simulink model "generic_src"  (Simulink 10.3)
settings: Solver=ode45  StartTime=0.0  StopTime=inf  RelTol=1e-3  EnableMultiTasking=on
undefined symbols (not defined in the file or in its folder): Area_Front, Area_Rear, ay_max_off, ay_max_on, ay_per_mu_max_off, ay_per_mu_max_on, Brake_ratio, brake_valve_ctrl_kP, cat1mode1_higher, cat1mode1_lower, cat1mode2_higher, cat1mode2_lower, cat1mode3_higher, cat1mode3_lower, cat2mode1_higher, cat2mode1_lower, cat2mode2_higher, cat2mode2_lower, cat2mode3_higher, cat2mode3_lower, delta_vel, diff_lock_fac, diff_lock_off, diff_lock_on, ESP_ctrl_kD, ESP_ctrl_kI, ESP_ctrl_kP, ESP_ctrl_restore_kI, ESP_min_throttle_fac, f_ax, f_slip, g, higherlimit_highvel, higherlimit_lowvel, highervel_fac, highervelocity_fac, InitialConditionForIntegrator, limit_acc, limit_selectlow, limit_starting, limit_vdiff, locktime_throttle, lowerlimit_highvel, lowerlimit_lowvel, lowervel_fac, lowervelocity_fac, min_throttle, MPS2KMPH, MSR_ctrl_kD, MSR_ctrl_kI, MSR_ctrl_kP, MSR_min_throttle_fac, PID_kP_sideslip, PID_kP_yawrate, RADpS2RpM, rBrake, RpM2RADpS, SH_SL_switch, sideslip_vel_corr, sidesplip_deviation_max ... (+35)
libraries: CarMaker4SL x137, simulink x57, simulink_extras x6
(part 7 of 12)

== system generic_src/CarMaker/IPG Vehicle/PowerTrain/PTControl Example/PTControl_In/CreateBus PTC_Cfg Gearbox8 ==
  In : Inport
  BusCreator : BusCreator  Inputs=38
  Demux : Demux  Outputs=38
      settings: DisplayOption=none
  Out : Outport  VectorParamsAs1DForOutWhenUnconnected=off
  wires:
  Demux/38 -> BusCreator/38  "PTC_Cfg Gearbox8 iBGear16"
  Demux/37 -> BusCreator/37  "PTC_Cfg Gearbox8 iBGear15"
  Demux/36 -> BusCreator/36  "PTC_Cfg Gearbox8 iBGear14"
  Demux/35 -> BusCreator/35  "PTC_Cfg Gearbox8 iBGear13"
  Demux/34 -> BusCreator/34  "PTC_Cfg Gearbox8 iBGear12"
  Demux/33 -> BusCreator/33  "PTC_Cfg Gearbox8 iBGear11"
  Demux/32 -> BusCreator/32  "PTC_Cfg Gearbox8 iBGear10"
  Demux/31 -> BusCreator/31  "PTC_Cfg Gearbox8 iBGear9"
  Demux/30 -> BusCreator/30  "PTC_Cfg Gearbox8 iBGear8"
  Demux/29 -> BusCreator/29  "PTC_Cfg Gearbox8 iBGear7"
  Demux/28 -> BusCreator/28  "PTC_Cfg Gearbox8 iBGear6"
  Demux/27 -> BusCreator/27  "PTC_Cfg Gearbox8 iBGear5"
  Demux/26 -> BusCreator/26  "PTC_Cfg Gearbox8 iBGear4"
  Demux/25 -> BusCreator/25  "PTC_Cfg Gearbox8 iBGear3"
  Demux/24 -> BusCreator/24  "PTC_Cfg Gearbox8 iBGear2"
  Demux/23 -> BusCreator/23  "PTC_Cfg Gearbox8 iBGear1"
  Demux/22 -> BusCreator/22  "PTC_Cfg Gearbox8 iBGear0"
  Demux/21 -> BusCreator/21  "PTC_Cfg Gearbox8 nBGears"
  Demux/20 -> BusCreator/20  "PTC_Cfg Gearbox8 iFGear16"
  Demux/19 -> BusCreator/19  "PTC_Cfg Gearbox8 iFGear15"
  Demux/18 -> BusCreator/18  "PTC_Cfg Gearbox8 iFGear14"
  Demux/17 -> BusCreator/17  "PTC_Cfg Gearbox8 iFGear13"
  Demux/16 -> BusCreator/16  "PTC_Cfg Gearbox8 iFGear12"
  Demux/15 -> BusCreator/15  "PTC_Cfg Gearbox8 iFGear11"
  Demux/14 -> BusCreator/14  "PTC_Cfg Gearbox8 iFGear10"
  Demux/13 -> BusCreator/13  "PTC_Cfg Gearbox8 iFGear9"
  Demux/12 -> BusCreator/12  "PTC_Cfg Gearbox8 iFGear8"
  Demux/11 -> BusCreator/11  "PTC_Cfg Gearbox8 iFGear7"
  Demux/10 -> BusCreator/10  "PTC_Cfg Gearbox8 iFGear6"
  Demux/9 -> BusCreator/9  "PTC_Cfg Gearbox8 iFGear5"
  Demux/8 -> BusCreator/8  "PTC_Cfg Gearbox8 iFGear4"
  Demux/7 -> BusCreator/7  "PTC_Cfg Gearbox8 iFGear3"
  Demux/6 -> BusCreator/6  "PTC_Cfg Gearbox8 iFGear2"
  Demux/5 -> BusCreator/5  "PTC_Cfg Gearbox8 iFGear1"
  Demux/4 -> BusCreator/4  "PTC_Cfg Gearbox8 iFGear0"
  Demux/3 -> BusCreator/3  "PTC_Cfg Gearbox8 nFGears"
  Demux/2 -> BusCreator/2  "PTC_Cfg Gearbox8 ClKind"
  Demux/1 -> BusCreator/1  "PTC_Cfg Gearbox8 GBKind"
  BusCreator/1 -> Out/1
  In/1 -> Demux/1

== system generic_src/CarMaker/IPG Vehicle/PowerTrain/PTControl Example/PTControl_In/CreateBus PTC_Cfg Gearbox9 ==
  In : Inport
  BusCreator : BusCreator  Inputs=38
  Demux : Demux  Outputs=38
      settings: DisplayOption=none
  Out : Outport  VectorParamsAs1DForOutWhenUnconnected=off
  wires:
  Demux/38 -> BusCreator/38  "PTC_Cfg Gearbox9 iBGear16"
  Demux/37 -> BusCreator/37  "PTC_Cfg Gearbox9 iBGear15"
  Demux/36 -> BusCreator/36  "PTC_Cfg Gearbox9 iBGear14"
  Demux/35 -> BusCreator/35  "PTC_Cfg Gearbox9 iBGear13"
  Demux/34 -> BusCreator/34  "PTC_Cfg Gearbox9 iBGear12"
  Demux/33 -> BusCreator/33  "PTC_Cfg Gearbox9 iBGear11"
  Demux/32 -> BusCreator/32  "PTC_Cfg Gearbox9 iBGear10"
  Demux/31 -> BusCreator/31  "PTC_Cfg Gearbox9 iBGear9"
  Demux/30 -> BusCreator/30  "PTC_Cfg Gearbox9 iBGear8"
  Demux/29 -> BusCreator/29  "PTC_Cfg Gearbox9 iBGear7"
  Demux/28 -> BusCreator/28  "PTC_Cfg Gearbox9 iBGear6"
  Demux/27 -> BusCreator/27  "PTC_Cfg Gearbox9 iBGear5"
  Demux/26 -> BusCreator/26  "PTC_Cfg Gearbox9 iBGear4"
  Demux/25 -> BusCreator/25  "PTC_Cfg Gearbox9 iBGear3"
  Demux/24 -> BusCreator/24  "PTC_Cfg Gearbox9 iBGear2"
  Demux/23 -> BusCreator/23  "PTC_Cfg Gearbox9 iBGear1"
  Demux/22 -> BusCreator/22  "PTC_Cfg Gearbox9 iBGear0"
  Demux/21 -> BusCreator/21  "PTC_Cfg Gearbox9 nBGears"
  Demux/20 -> BusCreator/20  "PTC_Cfg Gearbox9 iFGear16"
  Demux/19 -> BusCreator/19  "PTC_Cfg Gearbox9 iFGear15"
  Demux/18 -> BusCreator/18  "PTC_Cfg Gearbox9 iFGear14"
  Demux/17 -> BusCreator/17  "PTC_Cfg Gearbox9 iFGear13"
  Demux/16 -> BusCreator/16  "PTC_Cfg Gearbox9 iFGear12"
  Demux/15 -> BusCreator/15  "PTC_Cfg Gearbox9 iFGear11"
  Demux/14 -> BusCreator/14  "PTC_Cfg Gearbox9 iFGear10"
  Demux/13 -> BusCreator/13  "PTC_Cfg Gearbox9 iFGear9"
  Demux/12 -> BusCreator/12  "PTC_Cfg Gearbox9 iFGear8"
  Demux/11 -> BusCreator/11  "PTC_Cfg Gearbox9 iFGear7"
  Demux/10 -> BusCreator/10  "PTC_Cfg Gearbox9 iFGear6"
  Demux/9 -> BusCreator/9  "PTC_Cfg Gearbox9 iFGear5"
  Demux/8 -> BusCreator/8  "PTC_Cfg Gearbox9 iFGear4"
  Demux/7 -> BusCreator/7  "PTC_Cfg Gearbox9 iFGear3"
  Demux/6 -> BusCreator/6  "PTC_Cfg Gearbox9 iFGear2"
  Demux/5 -> BusCreator/5  "PTC_Cfg Gearbox9 iFGear1"
  Demux/4 -> BusCreator/4  "PTC_Cfg Gearbox9 iFGear0"
  Demux/3 -> BusCreator/3  "PTC_Cfg Gearbox9 nFGears"
  Demux/2 -> BusCreator/2  "PTC_Cfg Gearbox9 ClKind"
  Demux/1 -> BusCreator/1  "PTC_Cfg Gearbox9 GBKind"
  BusCreator/1 -> Out/1
  In/1 -> Demux/1

== system generic_src/CarMaker/IPG Vehicle/PowerTrain/PTControl Example/PTControl_In/CreateBus PTC_Cfg ISG ==
  In : Inport
  BusCreator : BusCreator  Inputs=4
  Demux : Demux
      settings: DisplayOption=none
  Out : Outport  VectorParamsAs1DForOutWhenUnconnected=off
  wires:
  Demux/4 -> BusCreator/4  "PTC_Cfg ISG rotv_Gen_max"
  Demux/3 -> BusCreator/3  "PTC_Cfg ISG rotv_Mot_max"
  Demux/2 -> BusCreator/2  "PTC_Cfg ISG Ratio"
  Demux/1 -> BusCreator/1  "PTC_Cfg ISG Level"
  BusCreator/1 -> Out/1
  In/1 -> Demux/1

== system generic_src/CarMaker/IPG Vehicle/PowerTrain/PTControl Example/PTControl_In/CreateBus PTC_Cfg Misc ==
  In : Inport
  BusCreator : BusCreator  Inputs=14
  Demux : Demux  Outputs=14
      settings: DisplayOption=none
  Out : Outport  VectorParamsAs1DForOutWhenUnconnected=off
  wires:
  BusCreator/1 -> Out/1
  In/1 -> Demux/1
  Demux/4 -> BusCreator/4  "PTC_Cfg nClutch"
  Demux/11 -> BusCreator/11  "PTC_Cfg DriveSourcePos0"
  Demux/12 -> BusCreator/12  "PTC_Cfg DriveSourcePos1"
  Demux/14 -> BusCreator/14  "PTC_Cfg DriveSourcePos3"
  Demux/5 -> BusCreator/5  "PTC_Cfg nGearbox"
  Demux/2 -> BusCreator/2  "PTC_Cfg ClKind"
  Demux/10 -> BusCreator/10  "PTC_Cfg DL_iDiff_mean"
  Demux/9 -> BusCreator/9  "PTC_Cfg Aero_Frcx"
  Demux/1 -> BusCreator/1  "PTC_Cfg PTKind"
  Demux/8 -> BusCreator/8  "PTC_Cfg WheelRadius"
  Demux/13 -> BusCreator/13  "PTC_Cfg DriveSourcePos2"
  Demux/7 -> BusCreator/7  "PTC_Cfg Vehicle_nWheels"
  Demux/3 -> BusCreator/3  "PTC_Cfg nMotor"
  Demux/6 -> BusCreator/6  "PTC_Cfg nPlanetGear"

== system generic_src/CarMaker/IPG Vehicle/PowerTrain/PTControl Example/PTControl_In/CreateBus PTC_Cfg Motor ==
  In : Inport
  BusCreator : BusCreator  Inputs=48
  Demux : Demux  Outputs=48
      settings: DisplayOption=none
  Out : Outport  VectorParamsAs1DForOutWhenUnconnected=off
  wires:
  Demux/16 -> BusCreator/16  "PTC_Cfg Motor3 rotv_Gen_max"
  Demux/15 -> BusCreator/15  "PTC_Cfg Motor3 rotv_Mot_max"
  Demux/14 -> BusCreator/14  "PTC_Cfg Motor3 Ratio"
  Demux/13 -> BusCreator/13  "PTC_Cfg Motor3 Level"
  Demux/12 -> BusCreator/12  "PTC_Cfg Motor2 rotv_Gen_max"
  Demux/11 -> BusCreator/11  "PTC_Cfg Motor2 rotv_Mot_max"
  Demux/10 -> BusCreator/10  "PTC_Cfg Motor2 Ratio"
  Demux/9 -> BusCreator/9  "PTC_Cfg Motor2 Level"
  Demux/8 -> BusCreator/8  "PTC_Cfg Motor1 rotv_Gen_max"
  Demux/7 -> BusCreator/7  "PTC_Cfg Motor1 rotv_Mot_max"
  Demux/6 -> BusCreator/6  "PTC_Cfg Motor1 Ratio"
  Demux/5 -> BusCreator/5  "PTC_Cfg Motor1 Level"
  Demux/4 -> BusCreator/4  "PTC_Cfg Motor0 rotv_Gen_max"
  Demux/3 -> BusCreator/3  "PTC_Cfg Motor0 rotv_Mot_max"
  Demux/2 -> BusCreator/2  "PTC_Cfg Motor0 Ratio"
  Demux/1 -> BusCreator/1  "PTC_Cfg Motor0 Level"
  BusCreator/1 -> Out/1
  In/1 -> Demux/1
  Demux/17 -> BusCreator/17  "PTC_Cfg Motor4 Level"
  Demux/18 -> BusCreator/18  "PTC_Cfg Motor4 Ratio"
  Demux/19 -> BusCreator/19  "PTC_Cfg Motor4 rotv_Mot_max"
  Demux/20 -> BusCreator/20  "PTC_Cfg Motor4 rotv_Gen_max"
  Demux/21 -> BusCreator/21  "PTC_Cfg Motor5 Level"
  Demux/22 -> BusCreator/22  "PTC_Cfg Motor5 Ratio"
  Demux/23 -> BusCreator/23  "PTC_Cfg Motor5 rotv_Mot_max"
  Demux/24 -> BusCreator/24  "PTC_Cfg Motor5 rotv_Gen_max"
  Demux/25 -> BusCreator/25  "PTC_Cfg Motor6 Level"
  Demux/26 -> BusCreator/26  "PTC_Cfg Motor6 Ratio"
  Demux/27 -> BusCreator/27  "PTC_Cfg Motor6 rotv_Mot_max"
  Demux/28 -> BusCreator/28  "PTC_Cfg Motor6 rotv_Gen_max"
  Demux/29 -> BusCreator/29  "PTC_Cfg Motor7 Level"
  Demux/30 -> BusCreator/30  "PTC_Cfg Motor7 Ratio"
  Demux/31 -> BusCreator/31  "PTC_Cfg Motor7 rotv_Mot_max"
  Demux/32 -> BusCreator/32  "PTC_Cfg Motor7 rotv_Gen_max"
  Demux/33 -> BusCreator/33  "PTC_Cfg Motor8 Level"
  Demux/34 -> BusCreator/34  "PTC_Cfg Motor8 Ratio"
  Demux/35 -> BusCreator/35  "PTC_Cfg Motor8 rotv_Mot_max"
  Demux/36 -> BusCreator/36  "PTC_Cfg Motor8 rotv_Gen_max"
  Demux/37 -> BusCreator/37  "PTC_Cfg Motor9 Level"
  Demux/38 -> BusCreator/38  "PTC_Cfg Motor9 Ratio"
  Demux/39 -> BusCreator/39  "PTC_Cfg Motor9 rotv_Mot_max"
  Demux/40 -> BusCreator/40  "PTC_Cfg Motor9 rotv_Gen_max"
  Demux/41 -> BusCreator/41  "PTC_Cfg Motor10 Level"
  Demux/42 -> BusCreator/42  "PTC_Cfg Motor10 Ratio"
  Demux/43 -> BusCreator/43  "PTC_Cfg Motor10 rotv_Mot_max"
  Demux/44 -> BusCreator/44  "PTC_Cfg Motor10 rotv_Gen_max"
  Demux/45 -> BusCreator/45  "PTC_Cfg Motor11 Level"
  Demux/46 -> BusCreator/46  "PTC_Cfg Motor11 Ratio"
  Demux/47 -> BusCreator/47  "PTC_Cfg Motor11 rotv_Mot_max"
  Demux/48 -> BusCreator/48  "PTC_Cfg Motor11 rotv_Gen_max"

== system generic_src/CarMaker/IPG Vehicle/PowerTrain/PTControl Example/PTControl_In/CreateBus PTC_Cfg PlanetGear ==
  In : Inport
  BusCreator : BusCreator  Inputs=1
  Demux : Demux  Outputs=1
      settings: DisplayOption=none
  Out : Outport  VectorParamsAs1DForOutWhenUnconnected=off
  wires:
  Demux/1 -> BusCreator/1  "PTC_Cfg PlanetGear0 Ratio"
  BusCreator/1 -> Out/1
  In/1 -> Demux/1

== system generic_src/CarMaker/IPG Vehicle/PowerTrain/TCU Example/PTTransmCU_In/CreateBus TCU ClutchIn0 ==
  In : Inport
  BusCreator : BusCreator  Inputs=7
  Demux : Demux  Outputs=7
      settings: DisplayOption=none
  Out : Outport  VectorParamsAs1DForOutWhenUnconnected=off
  wires:
  Demux/7 -> BusCreator/7  "TCU ClutchIn0 i_TrqIn2Out"
  Demux/6 -> BusCreator/6  "TCU ClutchIn0 Trq_out_trg"
  Demux/5 -> BusCreator/5  "TCU ClutchIn0 Trq_out"
  Demux/4 -> BusCreator/4  "TCU ClutchIn0 Trq_in"
  Demux/3 -> BusCreator/3  "TCU ClutchIn0 rotv_out_trg"
  Demux/2 -> BusCreator/2  "TCU ClutchIn0 rotv_out"
  Demux/1 -> BusCreator/1  "TCU ClutchIn0 rotv_in"
  BusCreator/1 -> Out/1
  In/1 -> Demux/1

== system generic_src/CarMaker/IPG Vehicle/PowerTrain/TCU Example/PTTransmCU_In/CreateBus TCU ClutchIn1 ==
  In : Inport
  BusCreator : BusCreator  Inputs=7
  Demux : Demux  Outputs=7
      settings: DisplayOption=none
  Out : Outport  VectorParamsAs1DForOutWhenUnconnected=off
  wires:
  Demux/7 -> BusCreator/7  "TCU ClutchIn1 i_TrqIn2Out"
  Demux/6 -> BusCreator/6  "TCU ClutchIn1 Trq_out_trg"
  Demux/5 -> BusCreator/5  "TCU ClutchIn1 Trq_out"
  Demux/4 -> BusCreator/4  "TCU ClutchIn1 Trq_in"
  Demux/3 -> BusCreator/3  "TCU ClutchIn1 rotv_out_trg"
  Demux/2 -> BusCreator/2  "TCU ClutchIn1 rotv_out"
  Demux/1 -> BusCreator/1  "TCU ClutchIn1 rotv_in"
  BusCreator/1 -> Out/1
  In/1 -> Demux/1

== system generic_src/CarMaker/IPG Vehicle/PowerTrain/TCU Example/PTTransmCU_In/CreateBus TCU ClutchIn10 ==
  In : Inport
  BusCreator : BusCreator  Inputs=7
  Demux : Demux  Outputs=7
      settings: DisplayOption=none
  Out : Outport  VectorParamsAs1DForOutWhenUnconnected=off
  wires:
  Demux/7 -> BusCreator/7  "TCU ClutchIn10 i_TrqIn2Out"
  Demux/6 -> BusCreator/6  "TCU ClutchIn10 Trq_out_trg"
  Demux/5 -> BusCreator/5  "TCU ClutchIn10 Trq_out"
  Demux/4 -> BusCreator/4  "TCU ClutchIn10 Trq_in"
  Demux/3 -> BusCreator/3  "TCU ClutchIn10 rotv_out_trg"
  Demux/2 -> BusCreator/2  "TCU ClutchIn10 rotv_out"
  Demux/1 -> BusCreator/1  "TCU ClutchIn10 rotv_in"
  BusCreator/1 -> Out/1
  In/1 -> Demux/1

== system generic_src/CarMaker/IPG Vehicle/PowerTrain/TCU Example/PTTransmCU_In/CreateBus TCU ClutchIn11 ==
  In : Inport
  BusCreator : BusCreator  Inputs=7
  Demux : Demux  Outputs=7
      settings: DisplayOption=none
  Out : Outport  VectorParamsAs1DForOutWhenUnconnected=off
  wires:
  Demux/7 -> BusCreator/7  "TCU ClutchIn10 i_TrqIn2Out"
  Demux/6 -> BusCreator/6  "TCU ClutchIn10 Trq_out_trg"
  Demux/5 -> BusCreator/5  "TCU ClutchIn10 Trq_out"
  Demux/4 -> BusCreator/4  "TCU ClutchIn10 Trq_in"
  Demux/3 -> BusCreator/3  "TCU ClutchIn10 rotv_out_trg"
  Demux/2 -> BusCreator/2  "TCU ClutchIn10 rotv_out"
  Demux/1 -> BusCreator/1  "TCU ClutchIn10 rotv_in"
  BusCreator/1 -> Out/1
  In/1 -> Demux/1

== system generic_src/CarMaker/IPG Vehicle/PowerTrain/TCU Example/PTTransmCU_In/CreateBus TCU ClutchIn2 ==
  In : Inport
  BusCreator : BusCreator  Inputs=7
  Demux : Demux  Outputs=7
      settings: DisplayOption=none
  Out : Outport  VectorParamsAs1DForOutWhenUnconnected=off
  wires:
  Demux/7 -> BusCreator/7  "TCU ClutchIn2 i_TrqIn2Out"
  Demux/6 -> BusCreator/6  "TCU ClutchIn2 Trq_out_trg"
  Demux/5 -> BusCreator/5  "TCU ClutchIn2 Trq_out"
  Demux/4 -> BusCreator/4  "TCU ClutchIn2 Trq_in"
  Demux/3 -> BusCreator/3  "TCU ClutchIn2 rotv_out_trg"
  Demux/2 -> BusCreator/2  "TCU ClutchIn2 rotv_out"
  Demux/1 -> BusCreator/1  "TCU ClutchIn2 rotv_in"
  BusCreator/1 -> Out/1
  In/1 -> Demux/1

== system generic_src/CarMaker/IPG Vehicle/PowerTrain/TCU Example/PTTransmCU_In/CreateBus TCU ClutchIn3 ==
  In : Inport
  BusCreator : BusCreator  Inputs=7
  Demux : Demux  Outputs=7
      settings: DisplayOption=none
  Out : Outport  VectorParamsAs1DForOutWhenUnconnected=off
  wires:
  Demux/7 -> BusCreator/7  "TCU ClutchIn3 i_TrqIn2Out"
  Demux/6 -> BusCreator/6  "TCU ClutchIn3 Trq_out_trg"
  Demux/5 -> BusCreator/5  "TCU ClutchIn3 Trq_out"
  Demux/4 -> BusCreator/4  "TCU ClutchIn3 Trq_in"
  Demux/3 -> BusCreator/3  "TCU ClutchIn3 rotv_out_trg"
  Demux/2 -> BusCreator/2  "TCU ClutchIn3 rotv_out"
  Demux/1 -> BusCreator/1  "TCU ClutchIn3 rotv_in"
  BusCreator/1 -> Out/1
  In/1 -> Demux/1

== system generic_src/CarMaker/IPG Vehicle/PowerTrain/TCU Example/PTTransmCU_In/CreateBus TCU ClutchIn4 ==
  In : Inport
  BusCreator : BusCreator  Inputs=7
  Demux : Demux  Outputs=7
      settings: DisplayOption=none
  Out : Outport  VectorParamsAs1DForOutWhenUnconnected=off
  wires:
  Demux/7 -> BusCreator/7  "TCU ClutchIn4 i_TrqIn2Out"
  Demux/6 -> BusCreator/6  "TCU ClutchIn4 Trq_out_trg"
  Demux/5 -> BusCreator/5  "TCU ClutchIn4 Trq_out"
  Demux/4 -> BusCreator/4  "TCU ClutchIn4 Trq_in"
  Demux/3 -> BusCreator/3  "TCU ClutchIn4 rotv_out_trg"
  Demux/2 -> BusCreator/2  "TCU ClutchIn4 rotv_out"
  Demux/1 -> BusCreator/1  "TCU ClutchIn4 rotv_in"
  BusCreator/1 -> Out/1
  In/1 -> Demux/1

== system generic_src/CarMaker/IPG Vehicle/PowerTrain/TCU Example/PTTransmCU_In/CreateBus TCU ClutchIn5 ==
  In : Inport
  BusCreator : BusCreator  Inputs=7
  Demux : Demux  Outputs=7
      settings: DisplayOption=none
  Out : Outport  VectorParamsAs1DForOutWhenUnconnected=off
  wires:
  Demux/7 -> BusCreator/7  "TCU ClutchIn5 i_TrqIn2Out"
  Demux/6 -> BusCreator/6  "TCU ClutchIn5 Trq_out_trg"
  Demux/5 -> BusCreator/5  "TCU ClutchIn5 Trq_out"
  Demux/4 -> BusCreator/4  "TCU ClutchIn5 Trq_in"
  Demux/3 -> BusCreator/3  "TCU ClutchIn5 rotv_out_trg"
  Demux/2 -> BusCreator/2  "TCU ClutchIn5 rotv_out"
  Demux/1 -> BusCreator/1  "TCU ClutchIn5 rotv_in"
  BusCreator/1 -> Out/1
  In/1 -> Demux/1

== system generic_src/CarMaker/IPG Vehicle/PowerTrain/TCU Example/PTTransmCU_In/CreateBus TCU ClutchIn6 ==
  In : Inport
  BusCreator : BusCreator  Inputs=7
  Demux : Demux  Outputs=7
      settings: DisplayOption=none
  Out : Outport  VectorParamsAs1DForOutWhenUnconnected=off
  wires:
  Demux/7 -> BusCreator/7  "TCU ClutchIn6 i_TrqIn2Out"
  Demux/6 -> BusCreator/6  "TCU ClutchIn6 Trq_out_trg"
  Demux/5 -> BusCreator/5  "TCU ClutchIn6 Trq_out"
  Demux/4 -> BusCreator/4  "TCU ClutchIn6 Trq_in"
  Demux/3 -> BusCreator/3  "TCU ClutchIn6 rotv_out_trg"
  Demux/2 -> BusCreator/2  "TCU ClutchIn6 rotv_out"
  Demux/1 -> BusCreator/1  "TCU ClutchIn6 rotv_in"
  BusCreator/1 -> Out/1
  In/1 -> Demux/1

== system generic_src/CarMaker/IPG Vehicle/PowerTrain/TCU Example/PTTransmCU_In/CreateBus TCU ClutchIn7 ==
  In : Inport
  BusCreator : BusCreator  Inputs=7
  Demux : Demux  Outputs=7
      settings: DisplayOption=none
  Out : Outport  VectorParamsAs1DForOutWhenUnconnected=off
  wires:
  Demux/7 -> BusCreator/7  "TCU ClutchIn7 i_TrqIn2Out"
  Demux/6 -> BusCreator/6  "TCU ClutchIn7 Trq_out_trg"
  Demux/5 -> BusCreator/5  "TCU ClutchIn7 Trq_out"
  Demux/4 -> BusCreator/4  "TCU ClutchIn7 Trq_in"
  Demux/3 -> BusCreator/3  "TCU ClutchIn7 rotv_out_trg"
  Demux/2 -> BusCreator/2  "TCU ClutchIn7 rotv_out"
  Demux/1 -> BusCreator/1  "TCU ClutchIn7 rotv_in"
  BusCreator/1 -> Out/1
  In/1 -> Demux/1

== system generic_src/CarMaker/IPG Vehicle/PowerTrain/TCU Example/PTTransmCU_In/CreateBus TCU ClutchIn8 ==
  In : Inport
  BusCreator : BusCreator  Inputs=7
  Demux : Demux  Outputs=7
      settings: DisplayOption=none
  Out : Outport  VectorParamsAs1DForOutWhenUnconnected=off
  wires:
  Demux/7 -> BusCreator/7  "TCU ClutchIn8 i_TrqIn2Out"
  Demux/6 -> BusCreator/6  "TCU ClutchIn8 Trq_out_trg"
  Demux/5 -> BusCreator/5  "TCU ClutchIn8 Trq_out"
  Demux/4 -> BusCreator/4  "TCU ClutchIn8 Trq_in"
  Demux/3 -> BusCreator/3  "TCU ClutchIn8 rotv_out_trg"
  Demux/2 -> BusCreator/2  "TCU ClutchIn8 rotv_out"
  Demux/1 -> BusCreator/1  "TCU ClutchIn8 rotv_in"
  BusCreator/1 -> Out/1
  In/1 -> Demux/1

== system generic_src/CarMaker/IPG Vehicle/PowerTrain/TCU Example/PTTransmCU_In/CreateBus TCU ClutchIn9 ==
  In : Inport
  BusCreator : BusCreator  Inputs=7
  Demux : Demux  Outputs=7
      settings: DisplayOption=none
  Out : Outport  VectorParamsAs1DForOutWhenUnconnected=off
  wires:
  Demux/7 -> BusCreator/7  "TCU ClutchIn9 i_TrqIn2Out"
  Demux/6 -> BusCreator/6  "TCU ClutchIn9 Trq_out_trg"
  Demux/5 -> BusCreator/5  "TCU ClutchIn9 Trq_out"
  Demux/4 -> BusCreator/4  "TCU ClutchIn9 Trq_in"
  Demux/3 -> BusCreator/3  "TCU ClutchIn9 rotv_out_trg"
  Demux/2 -> BusCreator/2  "TCU ClutchIn9 rotv_out"
  Demux/1 -> BusCreator/1  "TCU ClutchIn9 rotv_in"
  BusCreator/1 -> Out/1
  In/1 -> Demux/1

== system generic_src/CarMaker/IPG Vehicle/PowerTrain/TCU Example/PTTransmCU_In/CreateBus TCU ClutchOut0 ==
  In : Inport
  BusCreator : BusCreator  Inputs=1
  Demux : Demux  Outputs=1
      settings: DisplayOption=none
  Out : Outport  VectorParamsAs1DForOutWhenUnconnected=off
  wires:
  Demux/1 -> BusCreator/1  "TCU ClutchOut0 Pos"
  BusCreator/1 -> Out/1
  In/1 -> Demux/1

== system generic_src/CarMaker/IPG Vehicle/PowerTrain/TCU Example/PTTransmCU_In/CreateBus TCU ClutchOut1 ==
  In : Inport
  BusCreator : BusCreator  Inputs=1
  Demux : Demux  Outputs=1
      settings: DisplayOption=none
  Out : Outport  VectorParamsAs1DForOutWhenUnconnected=off
  wires:
  Demux/1 -> BusCreator/1  "TCU ClutchOut1 Pos"
  BusCreator/1 -> Out/1
  In/1 -> Demux/1

== system generic_src/CarMaker/IPG Vehicle/PowerTrain/TCU Example/PTTransmCU_In/CreateBus TCU ClutchOut10 ==
  In : Inport
  BusCreator : BusCreator  Inputs=1
  Demux : Demux  Outputs=1
      settings: DisplayOption=none
  Out : Outport  VectorParamsAs1DForOutWhenUnconnected=off
  wires:
  Demux/1 -> BusCreator/1  "TCU ClutchOut10 Pos"
  BusCreator/1 -> Out/1
  In/1 -> Demux/1

== system generic_src/CarMaker/IPG Vehicle/PowerTrain/TCU Example/PTTransmCU_In/CreateBus TCU ClutchOut11 ==
  In : Inport
  BusCreator : BusCreator  Inputs=1
  Demux : Demux  Outputs=1
      settings: DisplayOption=none
  Out : Outport  VectorParamsAs1DForOutWhenUnconnected=off
  wires:
  Demux/1 -> BusCreator/1  "TCU ClutchOut11 Pos"
  BusCreator/1 -> Out/1
  In/1 -> Demux/1

== system generic_src/CarMaker/IPG Vehicle/PowerTrain/TCU Example/PTTransmCU_In/CreateBus TCU ClutchOut2 ==
  In : Inport
  BusCreator : BusCreator  Inputs=1
  Demux : Demux  Outputs=1
      settings: DisplayOption=none
  Out : Outport  VectorParamsAs1DForOutWhenUnconnected=off
  wires:
  Demux/1 -> BusCreator/1  "TCU ClutchOut2 Pos"
  BusCreator/1 -> Out/1
  In/1 -> Demux/1

== system generic_src/CarMaker/IPG Vehicle/PowerTrain/TCU Example/PTTransmCU_In/CreateBus TCU ClutchOut3 ==
  In : Inport
  BusCreator : BusCreator  Inputs=1
  Demux : Demux  Outputs=1
      settings: DisplayOption=none
  Out : Outport  VectorParamsAs1DForOutWhenUnconnected=off
  wires:
  Demux/1 -> BusCreator/1  "TCU ClutchOut3 Pos"
  BusCreator/1 -> Out/1
  In/1 -> Demux/1

== system generic_src/CarMaker/IPG Vehicle/PowerTrain/TCU Example/PTTransmCU_In/CreateBus TCU ClutchOut4 ==
  In : Inport
  BusCreator : BusCreator  Inputs=1
  Demux : Demux  Outputs=1
      settings: DisplayOption=none
  Out : Outport  VectorParamsAs1DForOutWhenUnconnected=off
  wires:
  Demux/1 -> BusCreator/1  "TCU ClutchOut4 Pos"
  BusCreator/1 -> Out/1
  In/1 -> Demux/1

== system generic_src/CarMaker/IPG Vehicle/PowerTrain/TCU Example/PTTransmCU_In/CreateBus TCU ClutchOut5 ==
  In : Inport
  BusCreator : BusCreator  Inputs=1
  Demux : Demux  Outputs=1
      settings: DisplayOption=none
  Out : Outport  VectorParamsAs1DForOutWhenUnconnected=off
  wires:
  Demux/1 -> BusCreator/1  "TCU ClutchOut5 Pos"
  BusCreator/1 -> Out/1
  In/1 -> Demux/1

== system generic_src/CarMaker/IPG Vehicle/PowerTrain/TCU Example/PTTransmCU_In/CreateBus TCU ClutchOut6 ==
  In : Inport
  BusCreator : BusCreator  Inputs=1
  Demux : Demux  Outputs=1
      settings: DisplayOption=none
  Out : Outport  VectorParamsAs1DForOutWhenUnconnected=off
  wires:
  Demux/1 -> BusCreator/1  "TCU ClutchOut6 Pos"
  BusCreator/1 -> Out/1
  In/1 -> Demux/1

== system generic_src/CarMaker/IPG Vehicle/PowerTrain/TCU Example/PTTransmCU_In/CreateBus TCU ClutchOut7 ==
  In : Inport
  BusCreator : BusCreator  Inputs=1
  Demux : Demux  Outputs=1
      settings: DisplayOption=none
  Out : Outport  VectorParamsAs1DForOutWhenUnconnected=off
  wires:
  Demux/1 -> BusCreator/1  "TCU ClutchOut7 Pos"
  BusCreator/1 -> Out/1
  In/1 -> Demux/1

== system generic_src/CarMaker/IPG Vehicle/PowerTrain/TCU Example/PTTransmCU_In/CreateBus TCU ClutchOut8 ==
  In : Inport
  BusCreator : BusCreator  Inputs=1
  Demux : Demux  Outputs=1
      settings: DisplayOption=none
  Out : Outport  VectorParamsAs1DForOutWhenUnconnected=off
  wires:
  Demux/1 -> BusCreator/1  "TCU ClutchOut8 Pos"
  BusCreator/1 -> Out/1
  In/1 -> Demux/1

== system generic_src/CarMaker/IPG Vehicle/PowerTrain/TCU Example/PTTransmCU_In/CreateBus TCU ClutchOut9 ==
  In : Inport
  BusCreator : BusCreator  Inputs=1
  Demux : Demux  Outputs=1
      settings: DisplayOption=none
  Out : Outport  VectorParamsAs1DForOutWhenUnconnected=off
  wires:
  Demux/1 -> BusCreator/1  "TCU ClutchOut9 Pos"
  BusCreator/1 -> Out/1
  In/1 -> Demux/1

== system generic_src/CarMaker/IPG Vehicle/PowerTrain/TCU Example/PTTransmCU_In/CreateBus TCU GearboxIn0 ==
  In : Inport
  BusCreator : BusCreator  Inputs=23
  Demux : Demux  Outputs=23
      settings: DisplayOption=none
  Out : Outport  VectorParamsAs1DForOutWhenUnconnected=off
  wires:
  Demux/23 -> BusCreator/23  "TCU GearboxIn0 Clutch_dis i_TrqIn2Out"
  Demux/22 -> BusCreator/22  "TCU GearboxIn0 Clutch_dis Trq_out_trg"
  Demux/21 -> BusCreator/21  "TCU GearboxIn0 Clutch_dis Trq_out"
  Demux/20 -> BusCreator/20  "TCU GearboxIn0 Clutch_dis Trq_in"
  Demux/19 -> BusCreator/19  "TCU GearboxIn0 Clutch_dis rotv_out_trg"
  Demux/18 -> BusCreator/18  "TCU GearboxIn0 Clutch_dis rotv_out"
  Demux/17 -> BusCreator/17  "TCU GearboxIn0 Clutch_dis rotv_in"
  Demux/16 -> BusCreator/16  "TCU GearboxIn0 Clutch i_TrqIn2Out"
  Demux/15 -> BusCreator/15  "TCU GearboxIn0 Clutch Trq_out_trg"
  Demux/14 -> BusCreator/14  "TCU GearboxIn0 Clutch Trq_out"
  Demux/13 -> BusCreator/13  "TCU GearboxIn0 Clutch Trq_in"
  Demux/12 -> BusCreator/12  "TCU GearboxIn0 Clutch rotv_out_trg"
  Demux/11 -> BusCreator/11  "TCU GearboxIn0 Clutch rotv_out"
  Demux/10 -> BusCreator/10  "TCU GearboxIn0 Clutch rotv_in"
  Demux/9 -> BusCreator/9  "TCU GearboxIn0 Trq_out_trg"
  Demux/8 -> BusCreator/8  "TCU GearboxIn0 Trq_out"
  Demux/7 -> BusCreator/7  "TCU GearboxIn0 Trq_in"
  Demux/6 -> BusCreator/6  "TCU GearboxIn0 rotv_out"
  Demux/5 -> BusCreator/5  "TCU GearboxIn0 rotv_in_trg"
  Demux/4 -> BusCreator/4  "TCU GearboxIn0 rotv_in"
  Demux/3 -> BusCreator/3  "TCU GearboxIn0 i"
  Demux/2 -> BusCreator/2  "TCU GearboxIn0 GearNo_dis"
  Demux/1 -> BusCreator/1  "TCU GearboxIn0 GearNo"
  BusCreator/1 -> Out/1
  In/1 -> Demux/1

== system generic_src/CarMaker/IPG Vehicle/PowerTrain/TCU Example/PTTransmCU_In/CreateBus TCU GearboxIn1 ==
  In : Inport
  BusCreator : BusCreator  Inputs=23
  Demux : Demux  Outputs=23
      settings: DisplayOption=none
  Out : Outport  VectorParamsAs1DForOutWhenUnconnected=off
  wires:
  Demux/23 -> BusCreator/23  "TCU GearboxIn1 Clutch_dis i_TrqIn2Out"
  Demux/22 -> BusCreator/22  "TCU GearboxIn1 Clutch_dis Trq_out_trg"
  Demux/21 -> BusCreator/21  "TCU GearboxIn1 Clutch_dis Trq_out"
  Demux/20 -> BusCreator/20  "TCU GearboxIn1 Clutch_dis Trq_in"
  Demux/19 -> BusCreator/19  "TCU GearboxIn1 Clutch_dis rotv_out_trg"
  Demux/18 -> BusCreator/18  "TCU GearboxIn1 Clutch_dis rotv_out"
  Demux/17 -> BusCreator/17  "TCU GearboxIn1 Clutch_dis rotv_in"
  Demux/16 -> BusCreator/16  "TCU GearboxIn1 Clutch i_TrqIn2Out"
  Demux/15 -> BusCreator/15  "TCU GearboxIn1 Clutch Trq_out_trg"
  Demux/14 -> BusCreator/14  "TCU GearboxIn1 Clutch Trq_out"
  Demux/13 -> BusCreator/13  "TCU GearboxIn1 Clutch Trq_in"
  Demux/12 -> BusCreator/12  "TCU GearboxIn1 Clutch rotv_out_trg"
  Demux/11 -> BusCreator/11  "TCU GearboxIn1 Clutch rotv_out"
  Demux/10 -> BusCreator/10  "TCU GearboxIn1 Clutch rotv_in"
  Demux/9 -> BusCreator/9  "TCU GearboxIn1 Trq_out_trg"
  Demux/8 -> BusCreator/8  "TCU GearboxIn1 Trq_out"
  Demux/7 -> BusCreator/7  "TCU GearboxIn1 Trq_in"
  Demux/6 -> BusCreator/6  "TCU GearboxIn1 rotv_out"
  Demux/5 -> BusCreator/5  "TCU GearboxIn1 rotv_in_trg"
  Demux/4 -> BusCreator/4  "TCU GearboxIn1 rotv_in"
  Demux/3 -> BusCreator/3  "TCU GearboxIn1 i"
  Demux/2 -> BusCreator/2  "TCU GearboxIn1 GearNo_dis"
  Demux/1 -> BusCreator/1  "TCU GearboxIn1 GearNo"
  BusCreator/1 -> Out/1
  In/1 -> Demux/1

== system generic_src/CarMaker/IPG Vehicle/PowerTrain/TCU Example/PTTransmCU_In/CreateBus TCU GearboxIn10 ==
  In : Inport
  BusCreator : BusCreator  Inputs=23
  Demux : Demux  Outputs=23
      settings: DisplayOption=none
  Out : Outport  VectorParamsAs1DForOutWhenUnconnected=off
  wires:
  Demux/23 -> BusCreator/23  "TCU GearboxIn10 Clutch_dis i_TrqIn2Out"
  Demux/22 -> BusCreator/22  "TCU GearboxIn10 Clutch_dis Trq_out_trg"
  Demux/21 -> BusCreator/21  "TCU GearboxIn10 Clutch_dis Trq_out"
  Demux/20 -> BusCreator/20  "TCU GearboxIn10 Clutch_dis Trq_in"
  Demux/19 -> BusCreator/19  "TCU GearboxIn10 Clutch_dis rotv_out_trg"
  Demux/18 -> BusCreator/18  "TCU GearboxIn10 Clutch_dis rotv_out"
  Demux/17 -> BusCreator/17  "TCU GearboxIn10 Clutch_dis rotv_in"
  Demux/16 -> BusCreator/16  "TCU GearboxIn10 Clutch i_TrqIn2Out"
  Demux/15 -> BusCreator/15  "TCU GearboxIn10 Clutch Trq_out_trg"
  Demux/14 -> BusCreator/14  "TCU GearboxIn10 Clutch Trq_out"
  Demux/13 -> BusCreator/13  "TCU GearboxIn10 Clutch Trq_in"
  Demux/12 -> BusCreator/12  "TCU GearboxIn10 Clutch rotv_out_trg"
  Demux/11 -> BusCreator/11  "TCU GearboxIn10 Clutch rotv_out"
  Demux/10 -> BusCreator/10  "TCU GearboxIn10 Clutch rotv_in"
  Demux/9 -> BusCreator/9  "TCU GearboxIn10 Trq_out_trg"
  Demux/8 -> BusCreator/8  "TCU GearboxIn10 Trq_out"
  Demux/7 -> BusCreator/7  "TCU GearboxIn10 Trq_in"
  Demux/6 -> BusCreator/6  "TCU GearboxIn10 rotv_out"
  Demux/5 -> BusCreator/5  "TCU GearboxIn10 rotv_in_trg"
  Demux/4 -> BusCreator/4  "TCU GearboxIn10 rotv_in"
  Demux/3 -> BusCreator/3  "TCU GearboxIn10 i"
  Demux/2 -> BusCreator/2  "TCU GearboxIn10 GearNo_dis"
  Demux/1 -> BusCreator/1  "TCU GearboxIn10 GearNo"
  BusCreator/1 -> Out/1
  In/1 -> Demux/1

== system generic_src/CarMaker/IPG Vehicle/PowerTrain/TCU Example/PTTransmCU_In/CreateBus TCU GearboxIn11 ==
  In : Inport
  BusCreator : BusCreator  Inputs=23
  Demux : Demux  Outputs=23
      settings: DisplayOption=none
  Out : Outport  VectorParamsAs1DForOutWhenUnconnected=off
  wires:
  Demux/23 -> BusCreator/23  "TCU GearboxIn11 Clutch_dis i_TrqIn2Out"
  Demux/22 -> BusCreator/22  "TCU GearboxIn11 Clutch_dis Trq_out_trg"
  Demux/21 -> BusCreator/21  "TCU GearboxIn11 Clutch_dis Trq_out"
  Demux/20 -> BusCreator/20  "TCU GearboxIn11 Clutch_dis Trq_in"
  Demux/19 -> BusCreator/19  "TCU GearboxIn11 Clutch_dis rotv_out_trg"
  Demux/18 -> BusCreator/18  "TCU GearboxIn11 Clutch_dis rotv_out"
  Demux/17 -> BusCreator/17  "TCU GearboxIn11 Clutch_dis rotv_in"
  Demux/16 -> BusCreator/16  "TCU GearboxIn11 Clutch i_TrqIn2Out"
  Demux/15 -> BusCreator/15  "TCU GearboxIn11 Clutch Trq_out_trg"
  Demux/14 -> BusCreator/14  "TCU GearboxIn11 Clutch Trq_out"
  Demux/13 -> BusCreator/13  "TCU GearboxIn11 Clutch Trq_in"
  Demux/12 -> BusCreator/12  "TCU GearboxIn11 Clutch rotv_out_trg"
  Demux/11 -> BusCreator/11  "TCU GearboxIn11 Clutch rotv_out"
  Demux/10 -> BusCreator/10  "TCU GearboxIn11 Clutch rotv_in"
  Demux/9 -> BusCreator/9  "TCU GearboxIn11 Trq_out_trg"
  Demux/8 -> BusCreator/8  "TCU GearboxIn11 Trq_out"
  Demux/7 -> BusCreator/7  "TCU GearboxIn11 Trq_in"
  Demux/6 -> BusCreator/6  "TCU GearboxIn11 rotv_out"
  Demux/5 -> BusCreator/5  "TCU GearboxIn11 rotv_in_trg"
  Demux/4 -> BusCreator/4  "TCU GearboxIn11 rotv_in"
  Demux/3 -> BusCreator/3  "TCU GearboxIn11 i"
  Demux/2 -> BusCreator/2  "TCU GearboxIn11 GearNo_dis"
  Demux/1 -> BusCreator/1  "TCU GearboxIn11 GearNo"
  BusCreator/1 -> Out/1
  In/1 -> Demux/1

== system generic_src/CarMaker/IPG Vehicle/PowerTrain/TCU Example/PTTransmCU_In/CreateBus TCU GearboxIn2 ==
  In : Inport
  BusCreator : BusCreator  Inputs=23
  Demux : Demux  Outputs=23
      settings: DisplayOption=none
  Out : Outport  VectorParamsAs1DForOutWhenUnconnected=off
  wires:
  Demux/23 -> BusCreator/23  "TCU GearboxIn2 Clutch_dis i_TrqIn2Out"
  Demux/22 -> BusCreator/22  "TCU GearboxIn2 Clutch_dis Trq_out_trg"
  Demux/21 -> BusCreator/21  "TCU GearboxIn2 Clutch_dis Trq_out"
  Demux/20 -> BusCreator/20  "TCU GearboxIn2 Clutch_dis Trq_in"
  Demux/19 -> BusCreator/19  "TCU GearboxIn2 Clutch_dis rotv_out_trg"
  Demux/18 -> BusCreator/18  "TCU GearboxIn2 Clutch_dis rotv_out"
  Demux/17 -> BusCreator/17  "TCU GearboxIn2 Clutch_dis rotv_in"
  Demux/16 -> BusCreator/16  "TCU GearboxIn2 Clutch i_TrqIn2Out"
  Demux/15 -> BusCreator/15  "TCU GearboxIn2 Clutch Trq_out_trg"
  Demux/14 -> BusCreator/14  "TCU GearboxIn2 Clutch Trq_out"
  Demux/13 -> BusCreator/13  "TCU GearboxIn2 Clutch Trq_in"
  Demux/12 -> BusCreator/12  "TCU GearboxIn2 Clutch rotv_out_trg"
  Demux/11 -> BusCreator/11  "TCU GearboxIn2 Clutch rotv_out"
  Demux/10 -> BusCreator/10  "TCU GearboxIn2 Clutch rotv_in"
  Demux/9 -> BusCreator/9  "TCU GearboxIn2 Trq_out_trg"
  Demux/8 -> BusCreator/8  "TCU GearboxIn2 Trq_out"
  Demux/7 -> BusCreator/7  "TCU GearboxIn2 Trq_in"
  Demux/6 -> BusCreator/6  "TCU GearboxIn2 rotv_out"
  Demux/5 -> BusCreator/5  "TCU GearboxIn2 rotv_in_trg"
  Demux/4 -> BusCreator/4  "TCU GearboxIn2 rotv_in"
  Demux/3 -> BusCreator/3  "TCU GearboxIn2 i"
  Demux/2 -> BusCreator/2  "TCU GearboxIn2 GearNo_dis"
  Demux/1 -> BusCreator/1  "TCU GearboxIn2 GearNo"
  BusCreator/1 -> Out/1
  In/1 -> Demux/1

== system generic_src/CarMaker/IPG Vehicle/PowerTrain/TCU Example/PTTransmCU_In/CreateBus TCU GearboxIn3 ==
  In : Inport
  BusCreator : BusCreator  Inputs=23
  Demux : Demux  Outputs=23
      settings: DisplayOption=none
  Out : Outport  VectorParamsAs1DForOutWhenUnconnected=off
  wires:
  Demux/23 -> BusCreator/23  "TCU GearboxIn3 Clutch_dis i_TrqIn2Out"
  Demux/22 -> BusCreator/22  "TCU GearboxIn3 Clutch_dis Trq_out_trg"
  Demux/21 -> BusCreator/21  "TCU GearboxIn3 Clutch_dis Trq_out"
  Demux/20 -> BusCreator/20  "TCU GearboxIn3 Clutch_dis Trq_in"
  Demux/19 -> BusCreator/19  "TCU GearboxIn3 Clutch_dis rotv_out_trg"
  Demux/18 -> BusCreator/18  "TCU GearboxIn3 Clutch_dis rotv_out"
  Demux/17 -> BusCreator/17  "TCU GearboxIn3 Clutch_dis rotv_in"
  Demux/16 -> BusCreator/16  "TCU GearboxIn3 Clutch i_TrqIn2Out"
  Demux/15 -> BusCreator/15  "TCU GearboxIn3 Clutch Trq_out_trg"
  Demux/14 -> BusCreator/14  "TCU GearboxIn3 Clutch Trq_out"
  Demux/13 -> BusCreator/13  "TCU GearboxIn3 Clutch Trq_in"
  Demux/12 -> BusCreator/12  "TCU GearboxIn3 Clutch rotv_out_trg"
  Demux/11 -> BusCreator/11  "TCU GearboxIn3 Clutch rotv_out"
  Demux/10 -> BusCreator/10  "TCU GearboxIn3 Clutch rotv_in"
  Demux/9 -> BusCreator/9  "TCU GearboxIn3 Trq_out_trg"
  Demux/8 -> BusCreator/8  "TCU GearboxIn3 Trq_out"
  Demux/7 -> BusCreator/7  "TCU GearboxIn3 Trq_in"
  Demux/6 -> BusCreator/6  "TCU GearboxIn3 rotv_out"
  Demux/5 -> BusCreator/5  "TCU GearboxIn3 rotv_in_trg"
  Demux/4 -> BusCreator/4  "TCU GearboxIn3 rotv_in"
  Demux/3 -> BusCreator/3  "TCU GearboxIn3 i"
  Demux/2 -> BusCreator/2  "TCU GearboxIn3 GearNo_dis"
  Demux/1 -> BusCreator/1  "TCU GearboxIn3 GearNo"
  BusCreator/1 -> Out/1
  In/1 -> Demux/1

== system generic_src/CarMaker/IPG Vehicle/PowerTrain/TCU Example/PTTransmCU_In/CreateBus TCU GearboxIn4 ==
  In : Inport
  BusCreator : BusCreator  Inputs=23
  Demux : Demux  Outputs=23
      settings: DisplayOption=none
  Out : Outport  VectorParamsAs1DForOutWhenUnconnected=off
  wires:
  Demux/23 -> BusCreator/23  "TCU GearboxIn4 Clutch_dis i_TrqIn2Out"
  Demux/22 -> BusCreator/22  "TCU GearboxIn4 Clutch_dis Trq_out_trg"
  Demux/21 -> BusCreator/21  "TCU GearboxIn4 Clutch_dis Trq_out"
  Demux/20 -> BusCreator/20  "TCU GearboxIn4 Clutch_dis Trq_in"
  Demux/19 -> BusCreator/19  "TCU GearboxIn4 Clutch_dis rotv_out_trg"
  Demux/18 -> BusCreator/18  "TCU GearboxIn4 Clutch_dis rotv_out"
  Demux/17 -> BusCreator/17  "TCU GearboxIn4 Clutch_dis rotv_in"
  Demux/16 -> BusCreator/16  "TCU GearboxIn4 Clutch i_TrqIn2Out"
  Demux/15 -> BusCreator/15  "TCU GearboxIn4 Clutch Trq_out_trg"
  Demux/14 -> BusCreator/14  "TCU GearboxIn4 Clutch Trq_out"
  Demux/13 -> BusCreator/13  "TCU GearboxIn4 Clutch Trq_in"
  Demux/12 -> BusCreator/12  "TCU GearboxIn4 Clutch rotv_out_trg"
  Demux/11 -> BusCreator/11  "TCU GearboxIn4 Clutch rotv_out"
  Demux/10 -> BusCreator/10  "TCU GearboxIn4 Clutch rotv_in"
  Demux/9 -> BusCreator/9  "TCU GearboxIn4 Trq_out_trg"
  Demux/8 -> BusCreator/8  "TCU GearboxIn4 Trq_out"
  Demux/7 -> BusCreator/7  "TCU GearboxIn4 Trq_in"
  Demux/6 -> BusCreator/6  "TCU GearboxIn4 rotv_out"
  Demux/5 -> BusCreator/5  "TCU GearboxIn4 rotv_in_trg"
  Demux/4 -> BusCreator/4  "TCU GearboxIn4 rotv_in"
  Demux/3 -> BusCreator/3  "TCU GearboxIn4 i"
  Demux/2 -> BusCreator/2  "TCU GearboxIn4 GearNo_dis"
  Demux/1 -> BusCreator/1  "TCU GearboxIn4 GearNo"
  BusCreator/1 -> Out/1
  In/1 -> Demux/1

== system generic_src/CarMaker/IPG Vehicle/PowerTrain/TCU Example/PTTransmCU_In/CreateBus TCU GearboxIn5 ==
  In : Inport
  BusCreator : BusCreator  Inputs=23
  Demux : Demux  Outputs=23
      settings: DisplayOption=none
  Out : Outport  VectorParamsAs1DForOutWhenUnconnected=off
  wires:
  Demux/23 -> BusCreator/23  "TCU GearboxIn5 Clutch_dis i_TrqIn2Out"
  Demux/22 -> BusCreator/22  "TCU GearboxIn5 Clutch_dis Trq_out_trg"
  Demux/21 -> BusCreator/21  "TCU GearboxIn5 Clutch_dis Trq_out"
  Demux/20 -> BusCreator/20  "TCU GearboxIn5 Clutch_dis Trq_in"
  Demux/19 -> BusCreator/19  "TCU GearboxIn5 Clutch_dis rotv_out_trg"
  Demux/18 -> BusCreator/18  "TCU GearboxIn5 Clutch_dis rotv_out"
  Demux/17 -> BusCreator/17  "TCU GearboxIn5 Clutch_dis rotv_in"
  Demux/16 -> BusCreator/16  "TCU GearboxIn5 Clutch i_TrqIn2Out"
  Demux/15 -> BusCreator/15  "TCU GearboxIn5 Clutch Trq_out_trg"
  Demux/14 -> BusCreator/14  "TCU GearboxIn5 Clutch Trq_out"
  Demux/13 -> BusCreator/13  "TCU GearboxIn5 Clutch Trq_in"
  Demux/12 -> BusCreator/12  "TCU GearboxIn5 Clutch rotv_out_trg"
  Demux/11 -> BusCreator/11  "TCU GearboxIn5 Clutch rotv_out"
  Demux/10 -> BusCreator/10  "TCU GearboxIn5 Clutch rotv_in"
  Demux/9 -> BusCreator/9  "TCU GearboxIn5 Trq_out_trg"
  Demux/8 -> BusCreator/8  "TCU GearboxIn5 Trq_out"
  Demux/7 -> BusCreator/7  "TCU GearboxIn5 Trq_in"
  Demux/6 -> BusCreator/6  "TCU GearboxIn5 rotv_out"
  Demux/5 -> BusCreator/5  "TCU GearboxIn5 rotv_in_trg"
  Demux/4 -> BusCreator/4  "TCU GearboxIn5 rotv_in"
  Demux/3 -> BusCreator/3  "TCU GearboxIn5 i"
  Demux/2 -> BusCreator/2  "TCU GearboxIn5 GearNo_dis"
  Demux/1 -> BusCreator/1  "TCU GearboxIn5 GearNo"
  BusCreator/1 -> Out/1
  In/1 -> Demux/1

== system generic_src/CarMaker/IPG Vehicle/PowerTrain/TCU Example/PTTransmCU_In/CreateBus TCU GearboxIn6 ==
  In : Inport
  BusCreator : BusCreator  Inputs=23
  Demux : Demux  Outputs=23
      settings: DisplayOption=none
  Out : Outport  VectorParamsAs1DForOutWhenUnconnected=off
  wires:
  Demux/23 -> BusCreator/23  "TCU GearboxIn6 Clutch_dis i_TrqIn2Out"
  Demux/22 -> BusCreator/22  "TCU GearboxIn6 Clutch_dis Trq_out_trg"
  Demux/21 -> BusCreator/21  "TCU GearboxIn6 Clutch_dis Trq_out"
  Demux/20 -> BusCreator/20  "TCU GearboxIn6 Clutch_dis Trq_in"
  Demux/19 -> BusCreator/19  "TCU GearboxIn6 Clutch_dis rotv_out_trg"
  Demux/18 -> BusCreator/18  "TCU GearboxIn6 Clutch_dis rotv_out"
  Demux/17 -> BusCreator/17  "TCU GearboxIn6 Clutch_dis rotv_in"
  Demux/16 -> BusCreator/16  "TCU GearboxIn6 Clutch i_TrqIn2Out"
  Demux/15 -> BusCreator/15  "TCU GearboxIn6 Clutch Trq_out_trg"
  Demux/14 -> BusCreator/14  "TCU GearboxIn6 Clutch Trq_out"
  Demux/13 -> BusCreator/13  "TCU GearboxIn6 Clutch Trq_in"
  Demux/12 -> BusCreator/12  "TCU GearboxIn6 Clutch rotv_out_trg"
  Demux/11 -> BusCreator/11  "TCU GearboxIn6 Clutch rotv_out"
  Demux/10 -> BusCreator/10  "TCU GearboxIn6 Clutch rotv_in"
  Demux/9 -> BusCreator/9  "TCU GearboxIn6 Trq_out_trg"
  Demux/8 -> BusCreator/8  "TCU GearboxIn6 Trq_out"
  Demux/7 -> BusCreator/7  "TCU GearboxIn6 Trq_in"
  Demux/6 -> BusCreator/6  "TCU GearboxIn6 rotv_out"
  Demux/5 -> BusCreator/5  "TCU GearboxIn6 rotv_in_trg"
  Demux/4 -> BusCreator/4  "TCU GearboxIn6 rotv_in"
  Demux/3 -> BusCreator/3  "TCU GearboxIn6 i"
  Demux/2 -> BusCreator/2  "TCU GearboxIn6 GearNo_dis"
  Demux/1 -> BusCreator/1  "TCU GearboxIn6 GearNo"
  BusCreator/1 -> Out/1
  In/1 -> Demux/1

== system generic_src/CarMaker/IPG Vehicle/PowerTrain/TCU Example/PTTransmCU_In/CreateBus TCU GearboxIn7 ==
  In : Inport
  BusCreator : BusCreator  Inputs=23
  Demux : Demux  Outputs=23
      settings: DisplayOption=none
  Out : Outport  VectorParamsAs1DForOutWhenUnconnected=off
  wires:
  Demux/23 -> BusCreator/23  "TCU GearboxIn7 Clutch_dis i_TrqIn2Out"
  Demux/22 -> BusCreator/22  "TCU GearboxIn7 Clutch_dis Trq_out_trg"
  Demux/21 -> BusCreator/21  "TCU GearboxIn7 Clutch_dis Trq_out"
  Demux/20 -> BusCreator/20  "TCU GearboxIn7 Clutch_dis Trq_in"
  Demux/19 -> BusCreator/19  "TCU GearboxIn7 Clutch_dis rotv_out_trg"
  Demux/18 -> BusCreator/18  "TCU GearboxIn7 Clutch_dis rotv_out"
  Demux/17 -> BusCreator/17  "TCU GearboxIn7 Clutch_dis rotv_in"
  Demux/16 -> BusCreator/16  "TCU GearboxIn7 Clutch i_TrqIn2Out"
  Demux/15 -> BusCreator/15  "TCU GearboxIn7 Clutch Trq_out_trg"
  Demux/14 -> BusCreator/14  "TCU GearboxIn7 Clutch Trq_out"
  Demux/13 -> BusCreator/13  "TCU GearboxIn7 Clutch Trq_in"
  Demux/12 -> BusCreator/12  "TCU GearboxIn7 Clutch rotv_out_trg"
  Demux/11 -> BusCreator/11  "TCU GearboxIn7 Clutch rotv_out"
  Demux/10 -> BusCreator/10  "TCU GearboxIn7 Clutch rotv_in"
  Demux/9 -> BusCreator/9  "TCU GearboxIn7 Trq_out_trg"
  Demux/8 -> BusCreator/8  "TCU GearboxIn7 Trq_out"
  Demux/7 -> BusCreator/7  "TCU GearboxIn7 Trq_in"
  Demux/6 -> BusCreator/6  "TCU GearboxIn7 rotv_out"
  Demux/5 -> BusCreator/5  "TCU GearboxIn7 rotv_in_trg"
  Demux/4 -> BusCreator/4  "TCU GearboxIn7 rotv_in"
  Demux/3 -> BusCreator/3  "TCU GearboxIn7 i"
  Demux/2 -> BusCreator/2  "TCU GearboxIn7 GearNo_dis"
  Demux/1 -> BusCreator/1  "TCU GearboxIn7 GearNo"
  BusCreator/1 -> Out/1
  In/1 -> Demux/1

== system generic_src/CarMaker/IPG Vehicle/PowerTrain/TCU Example/PTTransmCU_In/CreateBus TCU GearboxIn8 ==
  In : Inport
  BusCreator : BusCreator  Inputs=23
  Demux : Demux  Outputs=23
      settings: DisplayOption=none
  Out : Outport  VectorParamsAs1DForOutWhenUnconnected=off
  wires:
  Demux/23 -> BusCreator/23  "TCU GearboxIn8 Clutch_dis i_TrqIn2Out"
  Demux/22 -> BusCreator/22  "TCU GearboxIn8 Clutch_dis Trq_out_trg"
  Demux/21 -> BusCreator/21  "TCU GearboxIn8 Clutch_dis Trq_out"
  Demux/20 -> BusCreator/20  "TCU GearboxIn8 Clutch_dis Trq_in"
  Demux/19 -> BusCreator/19  "TCU GearboxIn8 Clutch_dis rotv_out_trg"
  Demux/18 -> BusCreator/18  "TCU GearboxIn8 Clutch_dis rotv_out"
  Demux/17 -> BusCreator/17  "TCU GearboxIn8 Clutch_dis rotv_in"
  Demux/16 -> BusCreator/16  "TCU GearboxIn8 Clutch i_TrqIn2Out"
  Demux/15 -> BusCreator/15  "TCU GearboxIn8 Clutch Trq_out_trg"
  Demux/14 -> BusCreator/14  "TCU GearboxIn8 Clutch Trq_out"
  Demux/13 -> BusCreator/13  "TCU GearboxIn8 Clutch Trq_in"
  Demux/12 -> BusCreator/12  "TCU GearboxIn8 Clutch rotv_out_trg"
  Demux/11 -> BusCreator/11  "TCU GearboxIn8 Clutch rotv_out"
  Demux/10 -> BusCreator/10  "TCU GearboxIn8 Clutch rotv_in"
  Demux/9 -> BusCreator/9  "TCU GearboxIn8 Trq_out_trg"
  Demux/8 -> BusCreator/8  "TCU GearboxIn8 Trq_out"
  Demux/7 -> BusCreator/7  "TCU GearboxIn8 Trq_in"
  Demux/6 -> BusCreator/6  "TCU GearboxIn8 rotv_out"
  Demux/5 -> BusCreator/5  "TCU GearboxIn8 rotv_in_trg"
  Demux/4 -> BusCreator/4  "TCU GearboxIn8 rotv_in"
  Demux/3 -> BusCreator/3  "TCU GearboxIn8 i"
  Demux/2 -> BusCreator/2  "TCU GearboxIn8 GearNo_dis"
  Demux/1 -> BusCreator/1  "TCU GearboxIn8 GearNo"
  BusCreator/1 -> Out/1
  In/1 -> Demux/1

== system generic_src/CarMaker/IPG Vehicle/PowerTrain/TCU Example/PTTransmCU_In/CreateBus TCU GearboxIn9 ==
  In : Inport
  BusCreator : BusCreator  Inputs=23
  Demux : Demux  Outputs=23
      settings: DisplayOption=none
  Out : Outport  VectorParamsAs1DForOutWhenUnconnected=off
  wires:
  Demux/23 -> BusCreator/23  "TCU GearboxIn9 Clutch_dis i_TrqIn2Out"
  Demux/22 -> BusCreator/22  "TCU GearboxIn9 Clutch_dis Trq_out_trg"
  Demux/21 -> BusCreator/21  "TCU GearboxIn9 Clutch_dis Trq_out"
  Demux/20 -> BusCreator/20  "TCU GearboxIn9 Clutch_dis Trq_in"
  Demux/19 -> BusCreator/19  "TCU GearboxIn9 Clutch_dis rotv_out_trg"
  Demux/18 -> BusCreator/18  "TCU GearboxIn9 Clutch_dis rotv_out"
  Demux/17 -> BusCreator/17  "TCU GearboxIn9 Clutch_dis rotv_in"
  Demux/16 -> BusCreator/16  "TCU GearboxIn9 Clutch i_TrqIn2Out"
  Demux/15 -> BusCreator/15  "TCU GearboxIn9 Clutch Trq_out_trg"
  Demux/14 -> BusCreator/14  "TCU GearboxIn9 Clutch Trq_out"
  Demux/13 -> BusCreator/13  "TCU GearboxIn9 Clutch Trq_in"
  Demux/12 -> BusCreator/12  "TCU GearboxIn9 Clutch rotv_out_trg"
  Demux/11 -> BusCreator/11  "TCU GearboxIn9 Clutch rotv_out"
  Demux/10 -> BusCreator/10  "TCU GearboxIn9 Clutch rotv_in"
  Demux/9 -> BusCreator/9  "TCU GearboxIn9 Trq_out_trg"
  Demux/8 -> BusCreator/8  "TCU GearboxIn9 Trq_out"
  Demux/7 -> BusCreator/7  "TCU GearboxIn9 Trq_in"
  Demux/6 -> BusCreator/6  "TCU GearboxIn9 rotv_out"
  Demux/5 -> BusCreator/5  "TCU GearboxIn9 rotv_in_trg"
  Demux/4 -> BusCreator/4  "TCU GearboxIn9 rotv_in"
  Demux/3 -> BusCreator/3  "TCU GearboxIn9 i"
  Demux/2 -> BusCreator/2  "TCU GearboxIn9 GearNo_dis"
  Demux/1 -> BusCreator/1  "TCU GearboxIn9 GearNo"
  BusCreator/1 -> Out/1
  In/1 -> Demux/1

== system generic_src/CarMaker/IPG Vehicle/PowerTrain/TCU Example/PTTransmCU_In/CreateBus TCU GearboxOut0 ==
  In : Inport
  BusCreator : BusCreator  Inputs=6
  Demux : Demux  Outputs=6
      settings: DisplayOption=none
  Out : Outport  VectorParamsAs1DForOutWhenUnconnected=off
  wires:
  Demux/6 -> BusCreator/6  "TCU GearboxOut0 Clutch_dis Pos"
  Demux/5 -> BusCreator/5  "TCU GearboxOut0 Clutch Pos"
  Demux/4 -> BusCreator/4  "TCU GearboxOut0 i_trg"
  Demux/3 -> BusCreator/3  "TCU GearboxOut0 set_ParkBrake"
  Demux/2 -> BusCreator/2  "TCU GearboxOut0 GearNoTrg_dis"
  Demux/1 -> BusCreator/1  "TCU GearboxOut0 GearNoTrg"
  BusCreator/1 -> Out/1
  In/1 -> Demux/1

== system generic_src/CarMaker/IPG Vehicle/PowerTrain/TCU Example/PTTransmCU_In/CreateBus TCU GearboxOut1 ==
  In : Inport
  BusCreator : BusCreator  Inputs=6
  Demux : Demux  Outputs=6
      settings: DisplayOption=none
  Out : Outport  VectorParamsAs1DForOutWhenUnconnected=off
  wires:
  Demux/6 -> BusCreator/6  "TCU GearboxOut1 Clutch_dis Pos"
  Demux/5 -> BusCreator/5  "TCU GearboxOut1 Clutch Pos"
  Demux/4 -> BusCreator/4  "TCU GearboxOut1 i_trg"
  Demux/3 -> BusCreator/3  "TCU GearboxOut1 set_ParkBrake"
  Demux/2 -> BusCreator/2  "TCU GearboxOut1 GearNoTrg_dis"
  Demux/1 -> BusCreator/1  "TCU GearboxOut1 GearNoTrg"
  BusCreator/1 -> Out/1
  In/1 -> Demux/1

== system generic_src/CarMaker/IPG Vehicle/PowerTrain/TCU Example/PTTransmCU_In/CreateBus TCU GearboxOut10 ==
  In : Inport
  BusCreator : BusCreator  Inputs=6
  Demux : Demux  Outputs=6
      settings: DisplayOption=none
  Out : Outport  VectorParamsAs1DForOutWhenUnconnected=off
  wires:
  Demux/6 -> BusCreator/6  "TCU GearboxOut10 Clutch_dis Pos"
  Demux/5 -> BusCreator/5  "TCU GearboxOut10 Clutch Pos"
  Demux/4 -> BusCreator/4  "TCU GearboxOut10 i_trg"
  Demux/3 -> BusCreator/3  "TCU GearboxOut10 set_ParkBrake"
  Demux/2 -> BusCreator/2  "TCU GearboxOut10 GearNoTrg_dis"
  Demux/1 -> BusCreator/1  "TCU GearboxOut10 GearNoTrg"
  BusCreator/1 -> Out/1
  In/1 -> Demux/1

== system generic_src/CarMaker/IPG Vehicle/PowerTrain/TCU Example/PTTransmCU_In/CreateBus TCU GearboxOut11 ==
  In : Inport
  BusCreator : BusCreator  Inputs=6
  Demux : Demux  Outputs=6
      settings: DisplayOption=none
  Out : Outport  VectorParamsAs1DForOutWhenUnconnected=off
  wires:
  Demux/6 -> BusCreator/6  "TCU GearboxOut11 Clutch_dis Pos"
  Demux/5 -> BusCreator/5  "TCU GearboxOut11 Clutch Pos"
  Demux/4 -> BusCreator/4  "TCU GearboxOut11 i_trg"
  Demux/3 -> BusCreator/3  "TCU GearboxOut11 set_ParkBrake"
  Demux/2 -> BusCreator/2  "TCU GearboxOut11 GearNoTrg_dis"
  Demux/1 -> BusCreator/1  "TCU GearboxOut11 GearNoTrg"
  BusCreator/1 -> Out/1
  In/1 -> Demux/1

== system generic_src/CarMaker/IPG Vehicle/PowerTrain/TCU Example/PTTransmCU_In/CreateBus TCU GearboxOut2 ==
  In : Inport
  BusCreator : BusCreator  Inputs=6
  Demux : Demux  Outputs=6
      settings: DisplayOption=none
  Out : Outport  VectorParamsAs1DForOutWhenUnconnected=off
  wires:
  Demux/6 -> BusCreator/6  "TCU GearboxOut2 Clutch_dis Pos"
  Demux/5 -> BusCreator/5  "TCU GearboxOut2 Clutch Pos"
  Demux/4 -> BusCreator/4  "TCU GearboxOut2 i_trg"
  Demux/3 -> BusCreator/3  "TCU GearboxOut2 set_ParkBrake"
  Demux/2 -> BusCreator/2  "TCU GearboxOut2 GearNoTrg_dis"
  Demux/1 -> BusCreator/1  "TCU GearboxOut2 GearNoTrg"
  BusCreator/1 -> Out/1
  In/1 -> Demux/1

== system generic_src/CarMaker/IPG Vehicle/PowerTrain/TCU Example/PTTransmCU_In/CreateBus TCU GearboxOut3 ==
  In : Inport
  BusCreator : BusCreator  Inputs=6
  Demux : Demux  Outputs=6
      settings: DisplayOption=none
  Out : Outport  VectorParamsAs1DForOutWhenUnconnected=off
  wires:
  Demux/6 -> BusCreator/6  "TCU GearboxOut3 Clutch_dis Pos"
  Demux/5 -> BusCreator/5  "TCU GearboxOut3 Clutch Pos"
  Demux/4 -> BusCreator/4  "TCU GearboxOut3 i_trg"
  Demux/3 -> BusCreator/3  "TCU GearboxOut3 set_ParkBrake"
  Demux/2 -> BusCreator/2  "TCU GearboxOut3 GearNoTrg_dis"
  Demux/1 -> BusCreator/1  "TCU GearboxOut3 GearNoTrg"
  BusCreator/1 -> Out/1
  In/1 -> Demux/1

== system generic_src/CarMaker/IPG Vehicle/PowerTrain/TCU Example/PTTransmCU_In/CreateBus TCU GearboxOut4 ==
  In : Inport
  BusCreator : BusCreator  Inputs=6
  Demux : Demux  Outputs=6
      settings: DisplayOption=none
  Out : Outport  VectorParamsAs1DForOutWhenUnconnected=off
  wires:
  Demux/6 -> BusCreator/6  "TCU GearboxOut4 Clutch_dis Pos"
  Demux/5 -> BusCreator/5  "TCU GearboxOut4 Clutch Pos"
  Demux/4 -> BusCreator/4  "TCU GearboxOut4 i_trg"
  Demux/3 -> BusCreator/3  "TCU GearboxOut4 set_ParkBrake"
  Demux/2 -> BusCreator/2  "TCU GearboxOut4 GearNoTrg_dis"
  Demux/1 -> BusCreator/1  "TCU GearboxOut4 GearNoTrg"
  BusCreator/1 -> Out/1
  In/1 -> Demux/1
